simulink model "Model1"  (R2023b)
settings: Solver=FixedStepAuto  StartTime=0.0  StopTime=20000  FixedStep=1  RelTol=1e-3
model workspace (MAT data in the model file):
  rho = 980
values from neighbouring files (symbols this model uses):
  A = 1    [Exercise1.m]
  Av_star = 0.001    [Exercise1.m]
  g = 9.8    [Exercise1.m]
  K = 0.01    [Exercise1.m]
  phi_o_star = 0.001    [Exercise1.m]
settings Model: Creator=arthu  LastModifiedBy=arthu

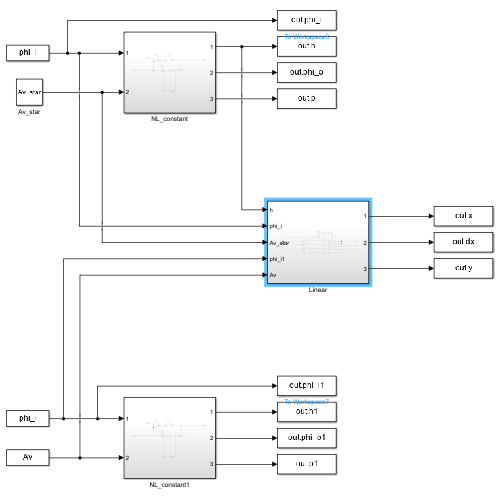
[thumbnail: Simulink's stored preview of the top-level diagram]
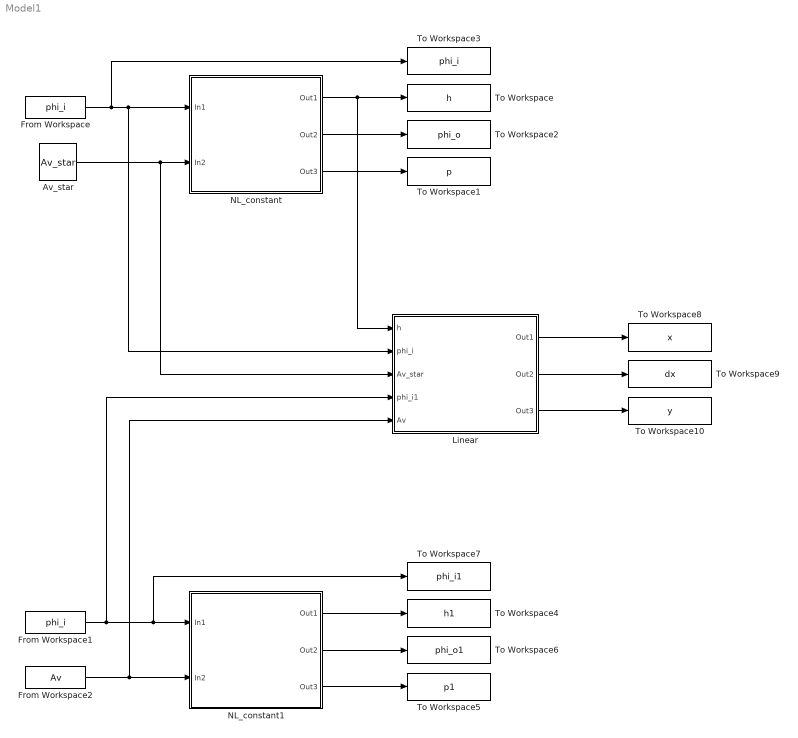
== system Model1 ==
  Av_star : Constant  Value=Av_star
  From Workspace : FromWorkspace  VariableName=phi_i
  From Workspace1 : FromWorkspace  VariableName=phi_i
  From Workspace2 : FromWorkspace  VariableName=Av
  Linear : Subsystem
  NL_constant : Subsystem
  NL_constant1 : Subsystem
  To Workspace : ToWorkspace  VariableName=h  SaveFormat=Timeseries  SampleTime=-1
  To Workspace1 : ToWorkspace  VariableName=p  SaveFormat=Timeseries  SampleTime=-1
  To Workspace10 : ToWorkspace  VariableName=y  SaveFormat=Timeseries  SampleTime=-1
  To Workspace2 : ToWorkspace  VariableName=phi_o  SaveFormat=Timeseries  SampleTime=-1
  To Workspace3 : ToWorkspace  VariableName=phi_i  SaveFormat=Timeseries  SampleTime=-1
  To Workspace4 : ToWorkspace  VariableName=h1  SaveFormat=Timeseries  SampleTime=-1
  To Workspace5 : ToWorkspace  VariableName=p1  SaveFormat=Timeseries  SampleTime=-1
  To Workspace6 : ToWorkspace  VariableName=phi_o1  SaveFormat=Timeseries  SampleTime=-1
  To Workspace7 : ToWorkspace  VariableName=phi_i1  SaveFormat=Timeseries  SampleTime=-1
  To Workspace8 : ToWorkspace  VariableName=x  SaveFormat=Timeseries  SampleTime=-1
  To Workspace9 : ToWorkspace  VariableName=dx  SaveFormat=Timeseries  SampleTime=-1
  wires:
  Av_star/1 -> Linear/3(Av_star), NL_constant/2(In2)
  NL_constant/2(Out2) -> To Workspace2/1
  NL_constant/3(Out3) -> To Workspace1/1
  From Workspace/1 -> To Workspace3/1, Linear/2(phi_i), NL_constant/1(In1)
  NL_constant1/2(Out2) -> To Workspace6/1
  NL_constant1/3(Out3) -> To Workspace5/1
  NL_constant1/1(Out1) -> To Workspace4/1
  From Workspace1/1 -> Linear/4(phi_i1), To Workspace7/1, NL_constant1/1(In1)
  From Workspace2/1 -> Linear/5(Av), NL_constant1/2(In2)
  NL_constant/1(Out1) -> To Workspace/1, Linear/1(h)
  Linear/1(Out1) -> To Workspace8/1
  Linear/2(Out2) -> To Workspace9/1
  Linear/3(Out3) -> To Workspace10/1

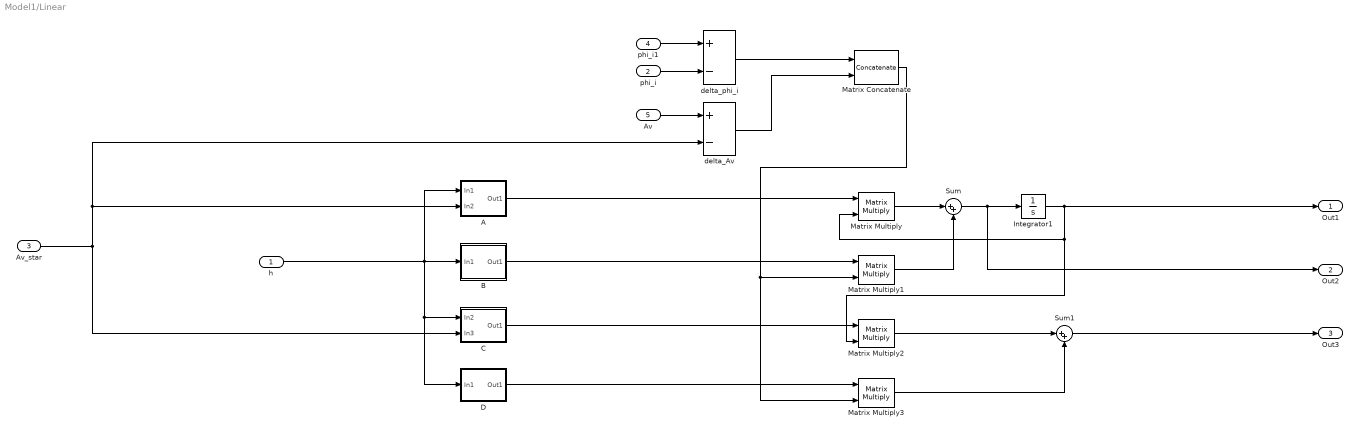
== system Model1/Linear ==
  h : Inport
  phi_i : Inport  Port=2
  Av_star : Inport  Port=3
  phi_i1 : Inport  Port=4
  Av : Inport  Port=5
  A : Subsystem
  B : Subsystem
  C : Subsystem
  D : Subsystem
  Integrator1 : Integrator
  Matrix Concatenate : Concatenate  Mode=Multidimensional array
  Matrix Multiply{,1..3} (4 alike) : Product  Multiplication=Matrix(*)
  Sum : Sum  Inputs=|++
  Sum1 : Sum  Inputs=|++
  delta_Av : Sum  Inputs=+-
  delta_phi_i : Sum  Inputs=+-
  Out1 : Outport
  Out2 : Outport  Port=2
  Out3 : Outport  Port=3
  wires:
  h/1 -> A/1(In1), B/1(In1), D/1(In1), C/1(In2)
  C/1(Out1) -> Matrix Multiply2/1
  Integrator1/1 -> Matrix Multiply/2, Matrix Multiply2/2, Out1/1
  phi_i/1 -> delta_phi_i/2
  Matrix Multiply2/1 -> Sum1/1
  delta_phi_i/1 -> Matrix Concatenate/1
  Matrix Multiply3/1 -> Sum1/2
  Matrix Concatenate/1 -> Matrix Multiply3/2, Matrix Multiply1/2
  Matrix Multiply1/1 -> Sum/2
  A/1(Out1) -> Matrix Multiply/1
  delta_Av/1 -> Matrix Concatenate/2
  B/1(Out1) -> Matrix Multiply1/1
  Matrix Multiply/1 -> Sum/1
  Av_star/1 -> C/2(In3), delta_Av/2, A/2(In2)
  phi_i1/1 -> delta_phi_i/1
  Sum1/1 -> Out3/1
  Av/1 -> delta_Av/1
  D/1(Out1) -> Matrix Multiply3/1
  Sum/1 -> Out2/1, Integrator1/1

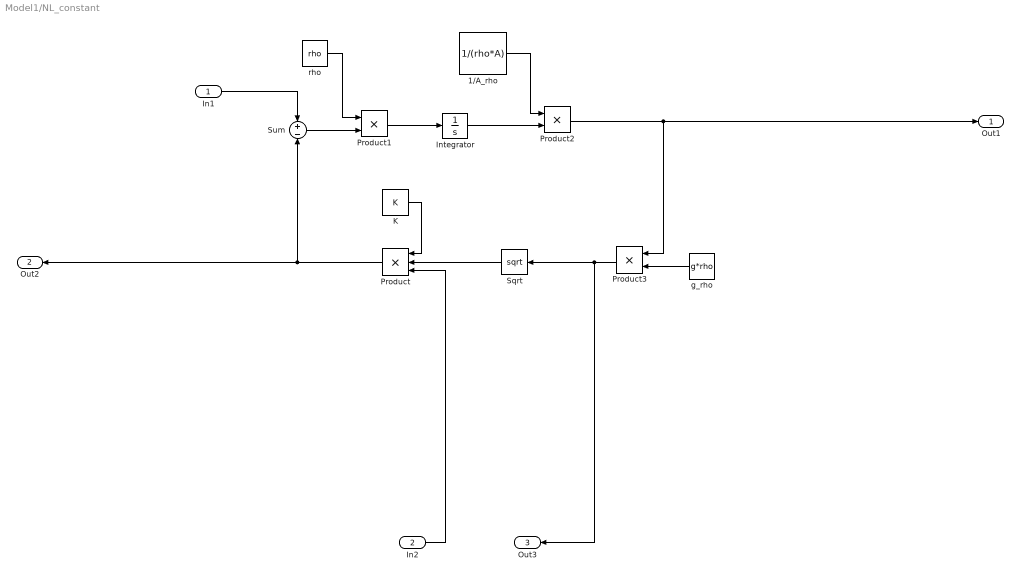
== system Model1/NL_constant ==
  In1 : Inport
  In2 : Inport  Port=2
  1/A_rho : Constant  Value=1/(rho*A)
  Integrator : Integrator  InitialCondition=A/g*(phi_o_star/(K*Av_star))^2
  K : Constant  Value=K
  Product : Product  Inputs=3
  Product1 : Product
  Product2 : Product
  Product3 : Product
  Sqrt : Sqrt
  Sum : Sum  Inputs=+-
  g_rho : Constant  Value=g*rho
  rho : Constant  Value=rho
  Out1 : Outport
  Out2 : Outport  Port=2
  Out3 : Outport  Port=3
  wires:
  Product3/1 -> Out3/1, Sqrt/1
  Integrator/1 -> Product2/2
  Sum/1 -> Product1/2
  rho/1 -> Product1/1
  Product/1 -> Out2/1, Sum/2
  In2/1 -> Product/3
  1/A_rho/1 -> Product2/1
  Product2/1 -> Out1/1, Product3/1
  Product1/1 -> Integrator/1
  K/1 -> Product/1
  Sqrt/1 -> Product/2
  g_rho/1 -> Product3/2
  In1/1 -> Sum/1

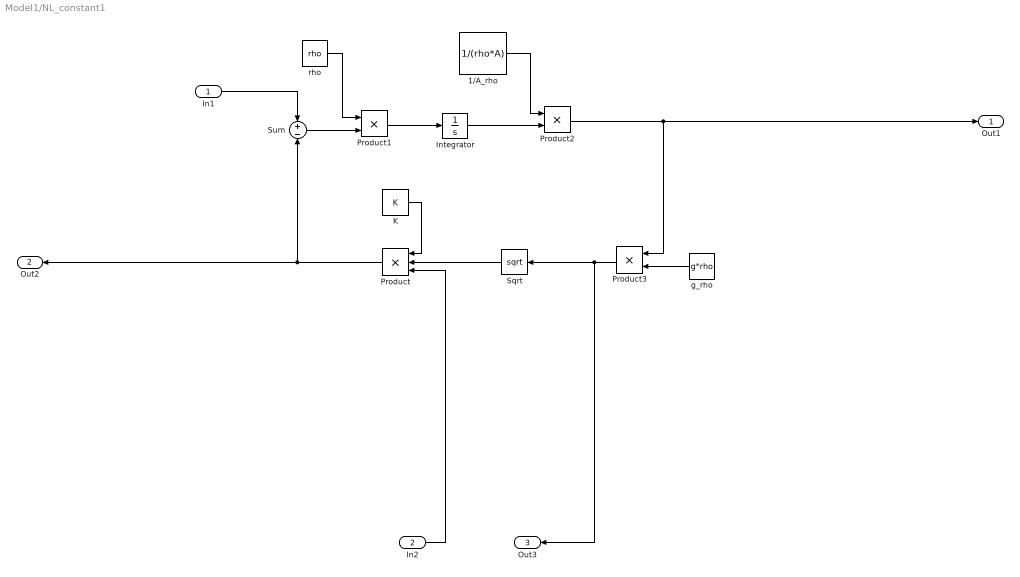
== system Model1/NL_constant1 ==
  In1 : Inport
  In2 : Inport  Port=2
  1/A_rho : Constant  Value=1/(rho*A)
  Integrator : Integrator  InitialCondition=A/g*(phi_o_star/(K*Av_star))^2
  K : Constant  Value=K
  Product : Product  Inputs=3
  Product1 : Product
  Product2 : Product
  Product3 : Product
  Sqrt : Sqrt
  Sum : Sum  Inputs=+-
  g_rho : Constant  Value=g*rho
  rho : Constant  Value=rho
  Out1 : Outport
  Out2 : Outport  Port=2
  Out3 : Outport  Port=3
  wires:
  Product3/1 -> Out3/1, Sqrt/1
  Integrator/1 -> Product2/2
  Sum/1 -> Product1/2
  rho/1 -> Product1/1
  Product/1 -> Out2/1, Sum/2
  In2/1 -> Product/3
  1/A_rho/1 -> Product2/1
  Product2/1 -> Out1/1, Product3/1
  Product1/1 -> Integrator/1
  K/1 -> Product/1
  Sqrt/1 -> Product/2
  g_rho/1 -> Product3/2
  In1/1 -> Sum/1

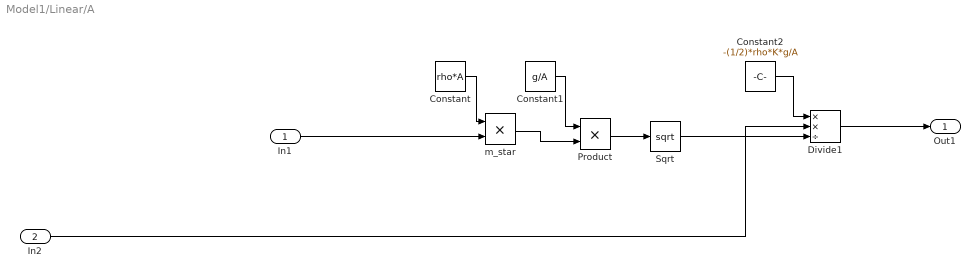
== system Model1/Linear/A ==
  In1 : Inport
  In2 : Inport  Port=2
  Constant : Constant  Value=rho*A
  Constant1 : Constant  Value=g/A
  Constant2 : Constant  Value=-(1/2)*rho*K*g/A
  Divide1 : Product  Inputs=**/
  Product : Product
  Sqrt : Sqrt
  m_star : Product
  Out1 : Outport
  wires:
  In2/1 -> Divide1/2
  m_star/1 -> Product/2
  Constant2/1 -> Divide1/1
  Constant1/1 -> Product/1
  Constant/1 -> m_star/1
  Sqrt/1 -> Divide1/3
  Product/1 -> Sqrt/1
  In1/1 -> m_star/2
  Divide1/1 -> Out1/1

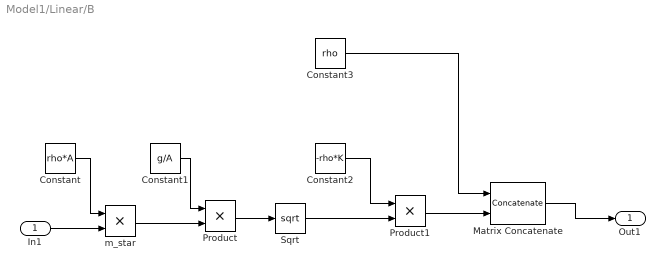
== system Model1/Linear/B ==
  In1 : Inport
  Constant : Constant  Value=rho*A
  Constant1 : Constant  Value=g/A
  Constant2 : Constant  Value=-rho*K
  Constant3 : Constant  Value=rho
  Matrix Concatenate : Concatenate  Mode=Multidimensional array  ConcatenateDimension=2
  Product : Product
  Product1 : Product
  Sqrt : Sqrt
  m_star : Product
  Out1 : Outport
  wires:
  Constant/1 -> m_star/1
  Product/1 -> Sqrt/1
  Constant1/1 -> Product/1
  m_star/1 -> Product/2
  In1/1 -> m_star/2
  Constant2/1 -> Product1/1
  Sqrt/1 -> Product1/2
  Constant3/1 -> Matrix Concatenate/1
  Product1/1 -> Matrix Concatenate/2
  Matrix Concatenate/1 -> Out1/1

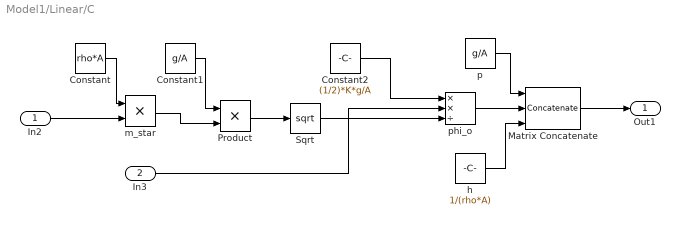
== system Model1/Linear/C ==
  In2 : Inport
  In3 : Inport  Port=2
  Constant : Constant  Value=rho*A
  Constant1 : Constant  Value=g/A
  Constant2 : Constant  Value=(1/2)*K*g/A
  Matrix Concatenate : Concatenate  NumInputs=3  Mode=Multidimensional array
  Product : Product
  Sqrt : Sqrt
  h : Constant  Value=1/(rho*A)
  m_star : Product
  p : Constant  Value=g/A
  phi_o : Product  Inputs=**/
  Out1 : Outport
  wires:
  In2/1 -> m_star/2
  Constant/1 -> m_star/1
  Product/1 -> Sqrt/1
  Sqrt/1 -> phi_o/3
  Constant1/1 -> Product/1
  m_star/1 -> Product/2
  Constant2/1 -> phi_o/1
  In3/1 -> phi_o/2
  Matrix Concatenate/1 -> Out1/1
  phi_o/1 -> Matrix Concatenate/2
  p/1 -> Matrix Concatenate/1
  h/1 -> Matrix Concatenate/3

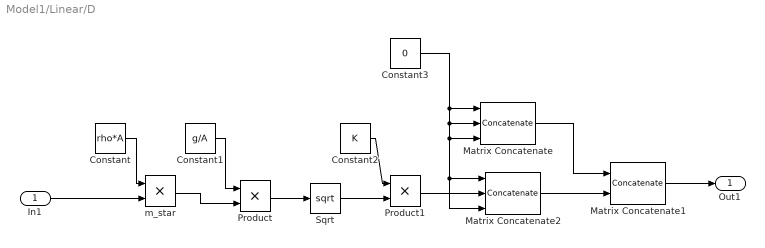
== system Model1/Linear/D ==
  In1 : Inport
  Constant : Constant  Value=rho*A
  Constant1 : Constant  Value=g/A
  Constant2 : Constant  Value=K
  Constant3 : Constant  Value=0
  Matrix Concatenate : Concatenate  NumInputs=3  Mode=Multidimensional array
  Matrix Concatenate1 : Concatenate  Mode=Multidimensional array  ConcatenateDimension=2
  Matrix Concatenate2 : Concatenate  NumInputs=3  Mode=Multidimensional array
  Product : Product
  Product1 : Product
  Sqrt : Sqrt
  m_star : Product
  Out1 : Outport
  wires:
  m_star/1 -> Product/2
  Constant1/1 -> Product/1
  Constant/1 -> m_star/1
  Product/1 -> Sqrt/1
  In1/1 -> m_star/2
  Constant2/1 -> Product1/1
  Sqrt/1 -> Product1/2
  Constant3/1 -> Matrix Concatenate/2, Matrix Concatenate/3, Matrix Concatenate2/1, Matrix Concatenate2/3, Matrix Concatenate/1
  Product1/1 -> Matrix Concatenate2/2
  Matrix Concatenate2/1 -> Matrix Concatenate1/2
  Matrix Concatenate/1 -> Matrix Concatenate1/1
  Matrix Concatenate1/1 -> Out1/1
